simulink model "EnvP"  (R2016b)
settings: Solver=VariableStepAuto  StartTime=0.0  StopTime=10.0  RelTol=1e-3
settings Model: Creator=jiakui  LastModifiedBy=jiakui

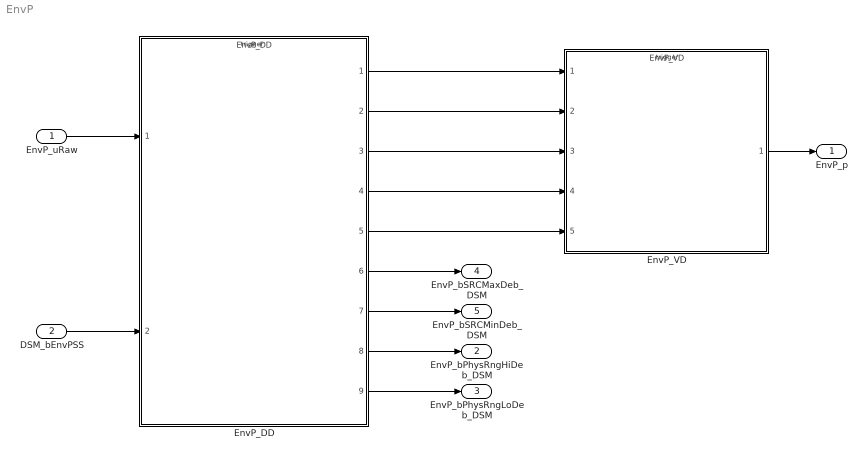
== system EnvP ==
  EnvP_uRaw : Inport  Tag=mv  Description=Sensor signal raw voltage  OutMin=0  OutMax=5000  OutDataTypeStr=Ad_mv
  DSM_bEnvPSS : Inport  Description=state of FId_EnvPSS  Port=2  OutMin=0  OutMax=1  OutDataTypeStr=boolean
  EnvP_DD : ModelReference  ModelNameDialog=EnvP_DD  SimulationMode=Normal  ModelReferenceVersion=1.9  TriggerPortName=function  TriggerPortTriggerType=function-call  TriggerPortStatesWhenEnabling=held
  EnvP_VD : ModelReference  ModelNameDialog=EnvP_VD  SimulationMode=Normal  ModelReferenceVersion=1.7  TriggerPortName=function  TriggerPortTriggerType=function-call  TriggerPortStatesWhenEnabling=held
  EnvP_p : Outport  Tag=kPa  Description=Barometric pressure  OutMin=0  OutMax=3276  OutDataTypeStr=AirPressure_kPa
  EnvP_bPhysRngHiDeb_DSM : Outport  Description=Physical-High of Environment pressure sensor  Port=2  OutMin=0  OutMax=1  OutDataTypeStr=boolean
  EnvP_bPhysRngLoDeb_DSM : Outport  Description=Physical-Low of Environment pressure sensor  Port=3  OutMin=0  OutMax=1  OutDataTypeStr=boolean
  EnvP_bSRCMaxDeb_DSM : Outport  Description=SRC-Max error of Environment pressure sensor  Port=4  OutMin=0  OutMax=1  OutDataTypeStr=boolean
  EnvP_bSRCMinDeb_DSM : Outport  Description=SRC-Min error of Environment pressure sensor  Port=5  OutMin=0  OutMax=1  OutDataTypeStr=boolean
  wires:
  EnvP_uRaw/1 -> EnvP_DD/1
  DSM_bEnvPSS/1 -> EnvP_DD/2
  EnvP_DD/1 -> EnvP_VD/1
  EnvP_DD/2 -> EnvP_VD/2
  EnvP_DD/3 -> EnvP_VD/3
  EnvP_DD/4 -> EnvP_VD/4
  EnvP_DD/5 -> EnvP_VD/5
  EnvP_VD/1 -> EnvP_p/1
  EnvP_DD/8 -> EnvP_bPhysRngHiDeb_DSM/1
  EnvP_DD/9 -> EnvP_bPhysRngLoDeb_DSM/1
  EnvP_DD/6 -> EnvP_bSRCMaxDeb_DSM/1
  EnvP_DD/7 -> EnvP_bSRCMinDeb_DSM/1
